simulink subsystem "balloon_drag_area"  (R2020a)
settings: Solver=VariableStepAuto  StartTime=0.0  StopTime=10.0  RelTol=1e-3
settings Model: Creator=Philip  LastModifiedBy=Philip

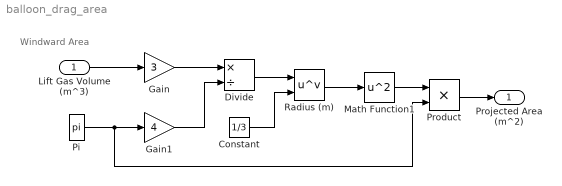
== system balloon_drag_area ==
  note: Windward Area
  Lift Gas Volume (m^3) : Inport
  Constant : Constant  Value=1/3
  Divide : Product  Inputs=*/
  Gain : Gain  Gain=3
  Gain1 : Gain  Gain=4
  Math Function1 : Math  Operator=square  SaturateOnIntegerOverflow=on
  Pi : Constant  Value=pi  OutDataTypeStr=Inherit: Inherit via back propagation
  Product : Product
  Radius (m) : Math  Operator=pow  SaturateOnIntegerOverflow=on
  Projected Area (m^2) : Outport
  wires:
  Constant/1 -> Radius (m)/2
  Lift Gas Volume (m^3)/1 -> Gain/1
  Divide/1 -> Radius (m)/1
  Radius (m)/1 -> Math Function1/1
  Math Function1/1 -> Product/1
  Product/1 -> Projected Area (m^2)/1
  Gain/1 -> Divide/1
  Gain1/1 -> Divide/2
  Pi/1 -> Gain1/1, Product/2
